simulink subsystem "DC_motor_gearbox"  (R2024b)
settings: Solver=VariableStepAuto  StartTime=0.0  StopTime=10.0  RelTol=1e-3
values from neighbouring files (symbols this model uses):
  Beq = 1.0459e-6    (= 1.0459e-06)    [Plant_ModelParameters.m]
  tau_sf = 0.0061    [Plant_ModelParameters.m]
undefined symbols (not defined in the file or in its folder): gbox, mld, mot, sens
settings Model: Creator=Federico Bergami  LastModifiedBy=Buton

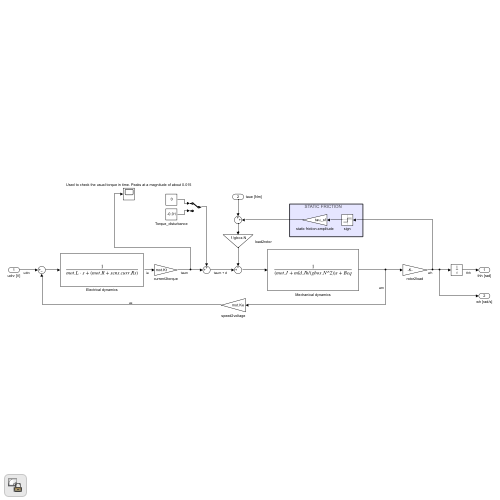
[thumbnail: Simulink's stored preview of the top-level diagram]
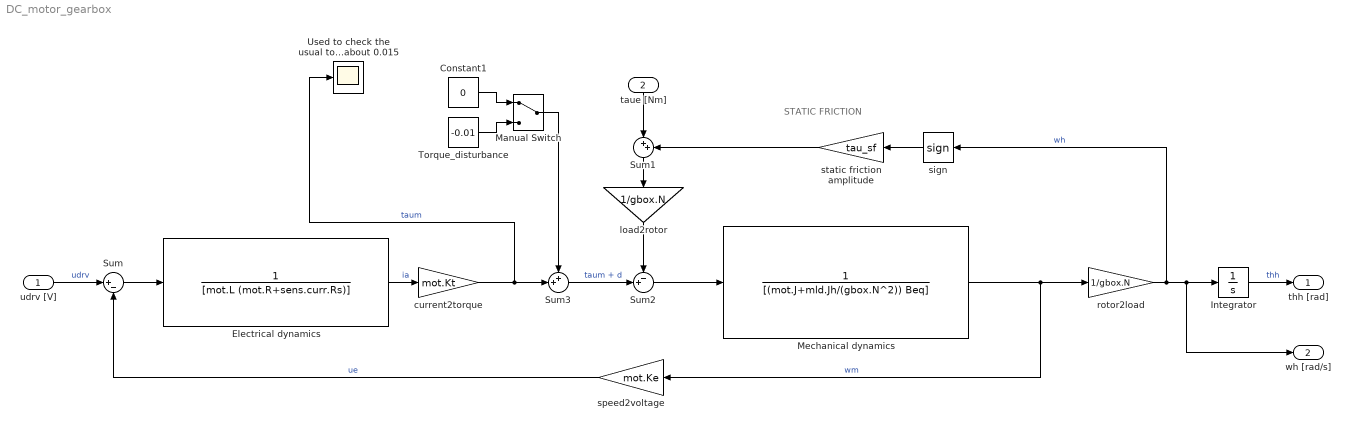
== system DC_motor_gearbox ==
  note: STATIC FRICTION
  udrv [V] : Inport
  taue [Nm] : Inport  Port=2
  Constant1 : Constant  Value=0
  Electrical dynamics : TransferFcn  Denominator=[mot.L (mot.R+sens.curr.Rs)]
  Integrator : Integrator  ZeroCross=off
  Manual Switch : ManualSwitch
  Mechanical dynamics : TransferFcn  Denominator=[(mot.J+mld.Jh/(gbox.N^2)) Beq]
  Sum : Sum  Inputs=|+-
  Sum1 : Sum  Inputs=|++
  Sum2 : Sum  Inputs=-+|
  Sum3 : Sum  Inputs=++|
  Torque_disturbance : Constant  Value=-0.01
  Used to check the usual torque in time. Peaks at a magnitude of about 0.015 : Scope
  current2torque : Gain  Gain=mot.Kt
  load2rotor : Gain  Gain=1/gbox.N
  rotor2load : Gain  Gain=1/gbox.N
  sign : Signum  ZeroCross=off
  speed2voltage : Gain  Gain=mot.Ke
  static friction amplitude : Gain  Gain=tau_sf
  thh [rad] : Outport
  wh [rad/s] : Outport  Port=2
  wires:
  taue [Nm]/1 -> Sum1/1
  Sum1/1 -> load2rotor/1
  load2rotor/1 -> Sum2/1
  udrv [V]/1 -> Sum/1  "udrv"
  current2torque/1 -> Sum3/2, Used to check the usual torque in time. Peaks at a magnitude of about 0.015/1  "taum"
  Sum/1 -> Electrical dynamics/1
  Electrical dynamics/1 -> current2torque/1  "ia"
  speed2voltage/1 -> Sum/2  "ue"
  Sum2/1 -> Mechanical dynamics/1
  Mechanical dynamics/1 -> speed2voltage/1, rotor2load/1  "wm"
  rotor2load/1 -> wh [rad/s]/1, Integrator/1, sign/1  "wh"
  Integrator/1 -> thh [rad]/1  "thh"
  sign/1 -> static friction amplitude/1
  static friction amplitude/1 -> Sum1/2
  Sum3/1 -> Sum2/2  "taum + d"
  Constant1/1 -> Manual Switch/1
  Manual Switch/1 -> Sum3/1
  Torque_disturbance/1 -> Manual Switch/2
